simulink model "chap3_5sim"  (Simulink 5.0)
settings: Solver=ode45  StartTime=0.0  StopTime=20  FixedStep=0.001  RelTol=1e-3
settings Model: LastModifiedBy=Administrator  ExtModeTrigMode=oneshot  ExtModeArmWhenConnect=off  LimitDataPoints=off  BooleanDataType=off

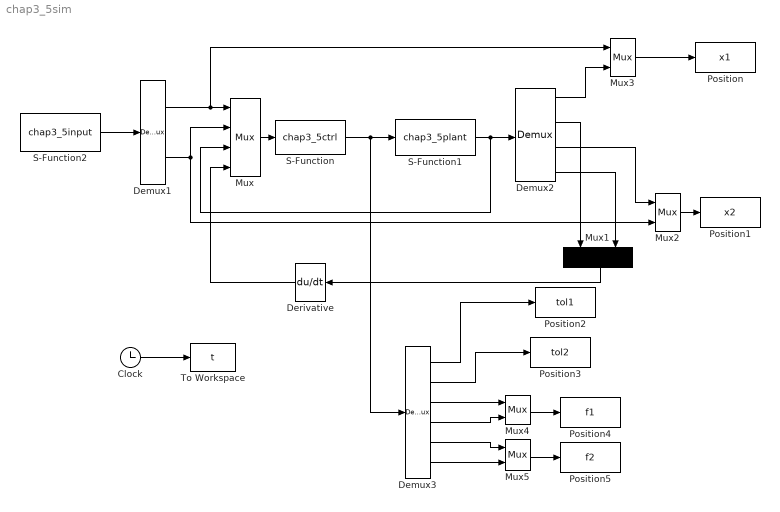
== system chap3_5sim ==
  Clock : Clock
      settings: Decimation=10
  Demux1 : Demux  Outputs=2
  Demux2 : Demux
  Demux3 : Demux  Outputs=6
  Derivative : Derivative  Orientation=left
  Mux : Mux
  Mux1 : Mux  Orientation=down  Inputs=2
  Mux{2..5} (4 alike) : Mux  Inputs=2
  Position : ToWorkspace  VariableName=x1  SampleTime=-1  SaveFormat=Array
  Position1 : ToWorkspace  VariableName=x2  SampleTime=-1  SaveFormat=Array
  Position2 : ToWorkspace  VariableName=tol1  SampleTime=-1  SaveFormat=Array
  Position3 : ToWorkspace  VariableName=tol2  SampleTime=-1  SaveFormat=Array
  Position4 : ToWorkspace  VariableName=f1  SampleTime=-1  SaveFormat=Array
  Position5 : ToWorkspace  VariableName=f2  SampleTime=-1  SaveFormat=Array
  S-Function : S-Function  FunctionName=chap3_5ctrl
  S-Function1 : S-Function  FunctionName=chap3_5plant
  S-Function2 : S-Function  FunctionName=chap3_5input
  To Workspace : ToWorkspace  VariableName=t  SampleTime=-1  SaveFormat=Array
  wires:
  Mux/1 -> S-Function/1
  Mux2/1 -> Position1/1
  Demux1/1 -> Mux3/1, Mux/1
  Mux3/1 -> Position/1
  Demux3/1 -> Position2/1
  Demux3/2 -> Position3/1
  S-Function/1 -> S-Function1/1, Demux3/1
  Demux1/2 -> Mux/2, Mux2/2
  Demux2/1 -> Mux3/2
  S-Function1/1 -> Demux2/1, Mux/3
  Demux2/3 -> Mux2/1
  S-Function2/1 -> Demux1/1
  Demux2/2 -> Mux1/1
  Demux2/4 -> Mux1/2
  Mux1/1 -> Derivative/1
  Derivative/1 -> Mux/4
  Demux3/3 -> Mux4/1
  Demux3/4 -> Mux4/2
  Demux3/6 -> Mux5/2
  Demux3/5 -> Mux5/1
  Mux5/1 -> Position5/1
  Mux4/1 -> Position4/1
  Clock/1 -> To Workspace/1
